simulink model "Problem15_model"  (R2020a)
settings: Solver=ode4  StartTime=0.0  StopTime=SIM_TIME  FixedStep=STEP_SIZE  RelTol=1e-3
values from neighbouring files (symbols this model uses):
  F = [tf([f1(1),f2(1)],1) ... (first row only)    [problem12.m]    (also in problem13.m; problem15.m = [tf([f2(1), f1(1), f0],1); problem16.m = [tf([f2(1), f1(1), f0],1); problem18.m = [tf([f2(1), f1(1), f0],1))
  f0 = kT * K_I    (= 225)    [problem15.m]    (also in problem16.m; problem18.m)
  f1 = @(q3) (1/2*K4*q3^2 - 1/2*m3*L3*q3)    [Problem7_9.m]    (also in problem12.m = kT * K_D ./ Jeff; problem13.m = kT * K_D ./ Jeff; problem15.m = kT * K_p; problem16.m = kT * K_p)
  f2 = @(q3) (m4*a4*q3)    [Problem7_9.m]    (also in problem12.m = kT * K_p ./ Jeff; problem13.m = kT * K_p ./ Jeff; problem15.m = kT * K_D; problem16.m = kT * K_D)
  G = 1/n^2 ./ Jeff    [problem13.m]    (also in problem15.m = tf([1/n^2, 0],1); problem16.m = tf([1/n^2, 0],1); problem18.m = tf([1/n^2, 0],1))
  N = [tf([n3(1), n2(1), n1(1), n0],1) ... (first row only)    [problem15.m]    (also in problem16.m; problem18.m)
  n = 53    [Problem7_9.m]    (also in Problem8_script.m = length(t); problem12.m; problem13.m; problem15.m)
  n0 = kT*K_I    (= 225)    [problem15.m]    (also in problem16.m; problem18.m)
  n1 = (feff + kT * K_D)./Jeff    [problem12.m]    (also in problem13.m; problem15.m = kT*K_p; problem16.m = kT*K_p; problem18.m = kT*K_p)
  n2 = kT * K_p ./ Jeff    [problem12.m]    (also in problem13.m; problem15.m = feff + kT*K_D; problem16.m = feff + kT*K_D; problem18.m = feff + kT*K_D)
  n3 = Jeff    [problem15.m]    (also in problem16.m; problem18.m)
  qr = [0.34, 0.34, 0.34, 0.34]    [problem12.m]    (also in problem13.m = [0.35, 0.35, 0.35, 0.35]; problem15.m = [0.35, 0.35, 0.35, 0.35]; problem16.m = [0.35, 0.35, 0.35, 0.35]; problem17.m = simout.qr)
  step_time = 0.01    [problem12.m]    (also in problem13.m; problem15.m; problem16.m)
  T_L = h    [problem13.m]    (also in problem15.m = zeros(4,1); problem16.m = zeros(4,1); problem17.m = abs(h); problem18.m = abs(h))
libraries: cstblocks x8
settings Model: Creator=Theis  LastModifiedBy=Theis

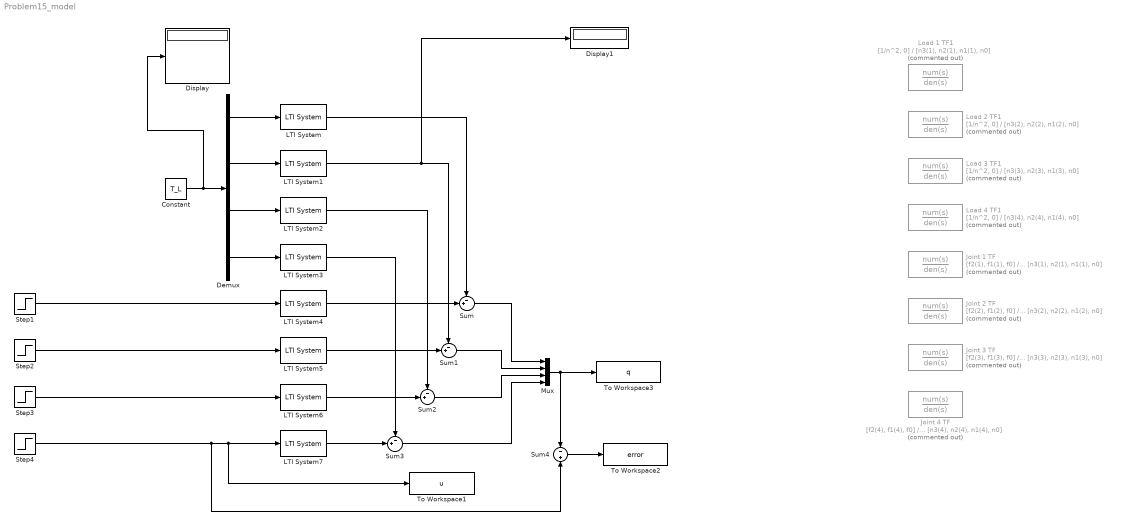
== system Problem15_model ==
  Constant : Constant  Value=T_L
  Demux : Demux
  Display : Display
  Display1 : Display
  Joint 1 TF : TransferFcn  Commented=on  Numerator=[f2(1), f1(1), f0]  Denominator=[n3(1), n2(1), n1(1), n0]
  Joint 2 TF : TransferFcn  Commented=on  Numerator=[f2(2), f1(2), f0]  Denominator=[n3(2), n2(2), n1(2), n0]
  Joint 3 TF : TransferFcn  Commented=on  Numerator=[f2(3), f1(3), f0]  Denominator=[n3(3), n2(3), n1(3), n0]
  Joint 4 TF : TransferFcn  Commented=on  Numerator=[f2(4), f1(4), f0]  Denominator=[n3(4), n2(4), n1(4), n0]
  LTI System : cstblocks/LTI System  sys=G/N(1)  IC=[]
  LTI System1 : cstblocks/LTI System  sys=G/N(2)  IC=[]
  LTI System2 : cstblocks/LTI System  sys=G/N(3)  IC=[]
  LTI System3 : cstblocks/LTI System  sys=G/N(4)  IC=[]
  LTI System4 : cstblocks/LTI System  sys=F(1)/N(1)  IC=[]
  LTI System5 : cstblocks/LTI System  sys=F(2)/N(2)  IC=[]
  LTI System6 : cstblocks/LTI System  sys=F(3)/N(3)  IC=[]
  LTI System7 : cstblocks/LTI System  sys=F(4)/N(4)  IC=[]
  Load 1 TF1 : TransferFcn  Commented=on  Numerator=[1/n^2, 0]  Denominator=[n3(1), n2(1), n1(1), n0]
  Load 2 TF1 : TransferFcn  Commented=on  Numerator=[1/n^2, 0]  Denominator=[n3(2), n2(2), n1(2), n0]
  Load 3 TF1 : TransferFcn  Commented=on  Numerator=[1/n^2, 0]  Denominator=[n3(3), n2(3), n1(3), n0]
  Load 4 TF1 : TransferFcn  Commented=on  Numerator=[1/n^2, 0]  Denominator=[n3(4), n2(4), n1(4), n0]
  Mux : Mux
  Step1 : Step  Time=step_time  After=qr(1)  SampleTime=0
  Step2 : Step  Time=step_time  After=qr(2)  SampleTime=0
  Step3 : Step  Time=step_time  After=qr(3)  SampleTime=0
  Step4 : Step  Time=step_time  After=qr(4)  SampleTime=0
  Sum{,1..3} (4 alike) : Sum  Inputs=-+|
  Sum4 : Sum  Inputs=-|+
  To Workspace1 : ToWorkspace  VariableName=u  SaveFormat=Timeseries  SampleTime=-1
  To Workspace2 : ToWorkspace  VariableName=error  SaveFormat=Timeseries  SampleTime=-1
  To Workspace3 : ToWorkspace  VariableName=q  SaveFormat=Timeseries  SampleTime=-1
  wires:
  Mux/1 -> To Workspace3/1, Sum4/1
  Sum/1 -> Mux/1
  Sum1/1 -> Mux/2
  Sum2/1 -> Mux/3
  Sum3/1 -> Mux/4
  Step3/1 -> LTI System6/1
  Step2/1 -> LTI System5/1
  Step1/1 -> LTI System4/1
  Step4/1 -> Sum4/2, To Workspace1/1, LTI System7/1
  Constant/1 -> Display/1, Demux/1
  LTI System4/1 -> Sum/2
  LTI System5/1 -> Sum1/2
  LTI System6/1 -> Sum2/2
  LTI System7/1 -> Sum3/2
  Demux/1 -> LTI System/1
  Demux/2 -> LTI System1/1
  Demux/3 -> LTI System2/1
  Demux/4 -> LTI System3/1
  LTI System3/1 -> Sum3/1
  LTI System2/1 -> Sum2/1
  LTI System1/1 -> Display1/1, Sum1/1
  LTI System/1 -> Sum/1
  Sum4/1 -> To Workspace2/1
